simulink model "HevP4TransmissionController"  (R2023b)
settings: Solver=FixedStepDiscrete  StartTime=0.0  StopTime=inf  FixedStep=0.01  RelTol=1e-3  EnableMultiTasking=on
model workspace (MAT data in the model file):
  Dn_Shft_Spd = Simulink.Parameter
  Dn_Shft_Spd.Value = reshape([10.8 10.8 36 36 25.2 25.2 61.2 61.2 39.6 39.6 93.6 93.6 54 54 126 126 68.4 68.4 176.4 176.4 31.6199307492 38.8199307492 42.4199307492 43.6199307492 44.3185789489 51.5185789489 55.1185789489 56.3185789489 53.5983603257 60.7983603257 64.3983603257 65.5983603257 66.2526076576 73.4526076576 77.0526076576 78.2526076576 84.5309649149 91.7309649149 95.3309649149 96.5309649149], [4 5 2])
  Dn_Shft_Spd.DataType = 'double'
  Dn_Shft_Spd.Complexity = 'real'
  Dn_Shft_Spd.Dimensions = [4 5 2]
  Pdl_Pos_Dn_bpt = Simulink.Parameter
  Pdl_Pos_Dn_bpt.Value = [0 0.6 0.9 1]
  Pdl_Pos_Dn_bpt.DataType = 'double'
  Pdl_Pos_Dn_bpt.Complexity = 'real'
  Pdl_Pos_Dn_bpt.Dimensions = [1 4]
  Pdl_Pos_Up_bpt = Simulink.Parameter
  Pdl_Pos_Up_bpt.Value = [0 0.25 0.9 1]
  Pdl_Pos_Up_bpt.DataType = 'double'
  Pdl_Pos_Up_bpt.Complexity = 'real'
  Pdl_Pos_Up_bpt.Dimensions = [1 4]
  Up_Shft_Spd = Simulink.Parameter
  Up_Shft_Spd.Value = reshape([18 18 43.2 43.2 32.4 32.4 68.4 68.4 46.8 46.8 100.8 100.8 61.2 61.2 133.2 133.2 75.6 75.6 183.6 183.6 35.6199307492 38.6199307492 46.4199307492 47.6199307492 48.3185789489 51.3185789489 59.1185789489 60.3185789489 57.5983603257 60.5983603257 68.3983603257 69.5983603257 70.2526076576 73.2526076576 81.0526076576 82.2526076576 88.5309649149 91.5309649149 99.3309649149 100.530964915], [4 5 2])
  Up_Shft_Spd.DataType = 'double'
  Up_Shft_Spd.Complexity = 'real'
  Up_Shft_Spd.Dimensions = [4 5 2]
libraries: autolibtranscontrolscommon x1
settings Model: DataDictionary=HevP4TransmissionController.sldd  ModifiedByFormat=The MathWorks, Inc.  Creator=The MathWorks, Inc.  LastModifiedBy=The MathWorks, Inc.
settings SolverCC: AlgebraicLoopSolver=TrustRegion  MaxZcPerStep=1
settings DataIOCC: SaveOutput=off  SaveTime=off  ReturnWorkspaceOutputs=off
settings OptimizationCC: DefaultParameterBehavior=Inlined  EnhancedBackFolding=on  PassReuseOutputArgsAs=Individual arguments  ZeroExternalMemoryAtStartup=off  ZeroInternalMemoryAtStartup=off  OptimizeBlockOrder=speed  DifferentSizesBufferReuse=on  OptimizationCustomize=off  EfficientTunableParamExpr=on
settings DebuggingCC: ParameterTunabilityLossMsg=error  UnconnectedInputMsg=warning  UnconnectedOutputMsg=warning  UnconnectedLineMsg=warning  SubsystemReferenceDiagnosticForUnitTest=warning  ArithmeticOperatorsInVariantConditions=warning
settings ModelReferenceCC: EnableRefExpFcnMdlSchedulingChecks=on
settings SFSimCC: SimUseLocalCustomCode=off  SimGenImportedTypeDefs=on  MATLABDynamicMemAlloc=off
settings RTWCC: Description=AUTOSAR  SystemTargetFile=autosar.tlc  GenCodeOnly=on  TemplateMakefile=ert_default_tmf  RTWUseLocalCustomCode=off  DLArmComputeVersion=19.05
settings CodeAppCC: ForceParamTrailComments=on  IgnoreCustomStorageClasses=off  OperatorAnnotations=on  SimulinkDataObjDesc=on  SFDataObjDesc=on  InsertBlockDesc=on
settings STFCustomTargetCC: MultiwordLength=256  ParMdlRefBuildCompliant=on  CompOptLevelCompliant=on  IncludeMdlTerminateFcn=off  CombineOutputUpdateFcns=on  SuppressErrorStatus=on  ERTCustomFileBanners=on  SupportNonFinite=off  SupportComplex=off  SupportContinuousTime=off  SupportNonInlinedSFcns=off  RemoveResetFunc=on  MATLABClassNameForMDSCustomization=Simulink.SoftwareTarget.ERTCustomization  AutosarCompliant=on  UseToolchainInfoCompliant=on  LookupTableObjectStructAxisOrder=2,1,3,4,...  LUTObjectStructOrderEvenSpacing=Size,Table,Breakpoints  SystemTargetFile=autosar.tlc
settings ERTTargetCC: TargetLangStandard=C99 (ISO)  ConcurrentExecutionCompliant=off  IncludeMdlTerminateFcn=off  SuppressErrorStatus=on  SupportNonFinite=off  SupportComplex=off  ModelStepFunctionPrototypeControlCompliant=off  CPPClassGenCompliant=off  AutosarCompliant=on  LookupTableObjectStructAxisOrder=2,1,3,4,...  LUTObjectStructOrderEvenSpacing=Size,Table,Breakpoints  InlinedParameterPlacement=NonHierarchical  ERTCustomFileTemplate=example_file_process.tlc

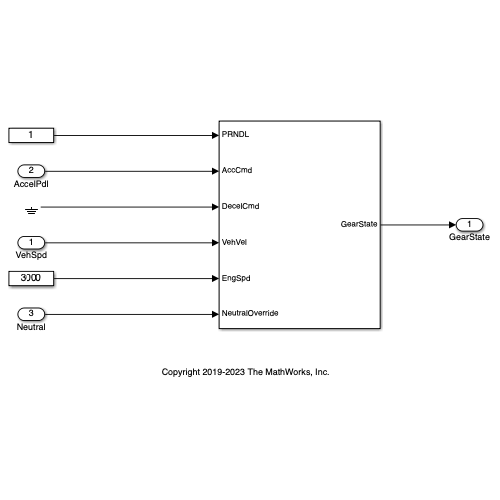
[thumbnail: Simulink's stored preview of the top-level diagram]
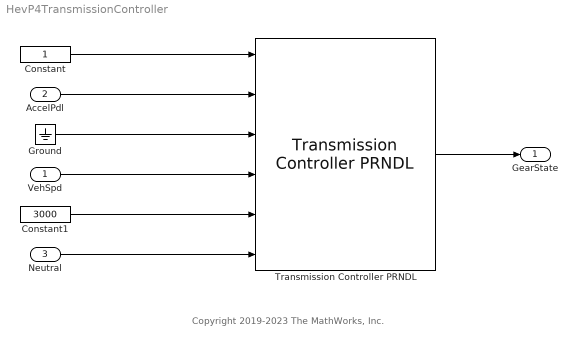
== system HevP4TransmissionController ==
  note: Copyright 2019-2023 The MathWorks, Inc.
  VehSpd : Inport  OutDataTypeStr=double  Unit=m/s  PortDimensions=1  SampleTime=[0.01,0]
  AccelPdl : Inport  Port=2  OutDataTypeStr=double  PortDimensions=1  SampleTime=[0.01,0]
  Neutral : Inport  Port=3  PortDimensions=1  SampleTime=[0.01,0]
  Constant : Constant
  Constant1 : Constant  Value=3000
  Ground : Ground
  Transmission Controller PRNDL : autolibtranscontrolscommon/Transmission Controller PRNDL  DriveMode=off  GearInit=1  LugSpd=1200  MinUpSpd=1000  tClutchUp=0.5  tClutchDn=0.5  tPark=120  VelUnit=km/hr  UpShSpd=Up_Shft_Spd  UpLdBpt=Pdl_Pos_Up_bpt  UpShBpt=1:5  UpPtBpt=[1 2]  DnShfSpd=Dn_Shft_Spd  DnShSpd=Dn_Shft_Spd  DnLdBpt=Pdl_Pos_Dn_bpt  DnShBpt=2:6  DnPtBpt=[1 2]  POFS=zeros(4,1)  GOFS=zeros(1,5)  Ngears=6  aMode=1
  GearState : Outport  PortDimensions=1  SampleTime=[0.01,0]  VectorParamsAs1DForOutWhenUnconnected=off
  wires:
  Transmission Controller PRNDL/1 -> GearState/1
  AccelPdl/1 -> Transmission Controller PRNDL/2
  VehSpd/1 -> Transmission Controller PRNDL/4
  Neutral/1 -> Transmission Controller PRNDL/6
  Ground/1 -> Transmission Controller PRNDL/3
  Constant/1 -> Transmission Controller PRNDL/1
  Constant1/1 -> Transmission Controller PRNDL/5
